simulink model "LightningModel"  (R2015a)
settings: Solver=ode23tb  StartTime=0.0  StopTime=0.04  RelTol=1e-3
libraries: powerlib x11, simulink x1
settings Model: CovSFcnEnable=off  Creator=Rodney Tan  LastModifiedBy=Rodney Tan
settings DebuggingCC: SolverPrmCheckMsg=warning

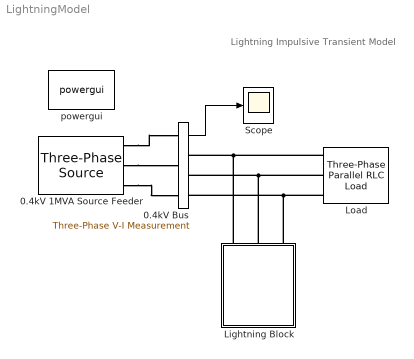
== system LightningModel ==
  note: Lightning Impulsive Transient Model
  0.4kV 1MVA Source Feeder : powerlib/Electrical Sources/Three-Phase Source  Voltage=0.4e3  PhaseAngle=0  Frequency=50  InternalConnection=Yg  SpecifyImpedance=on  Resistance=0.8929  Inductance=16.58e-3  ShortCircuitLevel=1e6  BaseVoltage=0.4e3  XRratio=7  BusType=swing  Pref=0  Qref=0  Qmin=-inf  Qmax=inf
  0.4kV Bus : powerlib/Measurements/Three-Phase V-I Measurement  VoltageMeasurement=phase-to-ground  SetLabelV=off  LabelV=Vabc  Vpu=off  VpuLL=off  CurrentMeasurement=no  SetLabelI=off  LabelI=Iabc  Ipu=off  Pbase=100e6  Vbase=500e3  OutputType=Complex  PhasorSimulation=off  PSBequivalent=0
  Lightning Block : Subsystem  mask(Lightning Model){mag=1e3, t1=0.012, R=1, L=1e-6}
      mask prompts: mag "Impulse Magnitude"; t1 "Impulse Start Time (s)"; R "Coupling Resistance (Ohms)"; L "Coupling Inductance (H)"
      mask help:
      | This lightning model simulate a 1.2/50us impulsive transient voltage defined by IEEE 1159.1 Standard. The impulsive transient is model by
      |
      | v = A*exp(-alpha*abs(t-t1))*u;
      |
      | where A is the impulse magnitude, t1 is the impulse start time, alpha is the damping factor of 14000 and u is the step function.
      mask DialogControl Container3 Prompt: Lightning Coupling
      mask Display: image('LightningBlock.jpg');
  Load : powerlib/Elements/Three-Phase Parallel RLC Load  LConnTagsString=A|B|C  Configuration=Y (grounded)  NominalVoltage=0.4e3  NominalFrequency=50  ActivePower=10e3  InductivePower=100  CapacitivePower=0  Measurements=None  LoadType=constant Z
  Scope : Scope
      settings: SampleTime=1/102400
  powergui : powerlib/powergui  Priority=1  SimulationMode=Continuous  SolverType=Tustin  SampleTime=50e-6  frequency=60  SPID=off  DisableSnubberDevices=off  DisableRonSwitches=off  DisableVfSwitches=off  SwTol=0  DisplayEquations=off  Interpol=off  methode=off  Ts=0  FunctionMessages=off  echomessages=off  HookPort=off  EnableUseOfTLC=off  x0status=blocks  frequencyindice=50  Pbase=100e6  ErrMax=1e-4  Iterations=50  UnitsV=kV  UnitsW=MW  buscounter=0  RestoreLinks=warning  ResistiveCurrentMeasurement=off  Frange=[0:2:500]  Ylog=off  Xlog=on  ShowGrid=off  save=off  variable=ZData  structure=0  ZoomFFT=off  StartTime=0.0  cycles=1  DisplayStyle=1  fundamental=60  FreqAxis=off  MaxFrequency=1000  frequencyindicesteady=1  RmsSteady=1  display=off
  wires:
  0.4kV Bus/1 -> Scope/1
  connections:
  0.4kV 1MVA Source Feeder/RConn2 -- 0.4kV Bus/LConn2
  0.4kV 1MVA Source Feeder/RConn3 -- 0.4kV Bus/LConn3
  0.4kV 1MVA Source Feeder/RConn1 -- 0.4kV Bus/LConn1
  Lightning Block/LConn2 -- Load/LConn2 -- 0.4kV Bus/RConn2
  Lightning Block/LConn1 -- Load/LConn1 -- 0.4kV Bus/RConn1
  Lightning Block/LConn3 -- Load/LConn3 -- 0.4kV Bus/RConn3

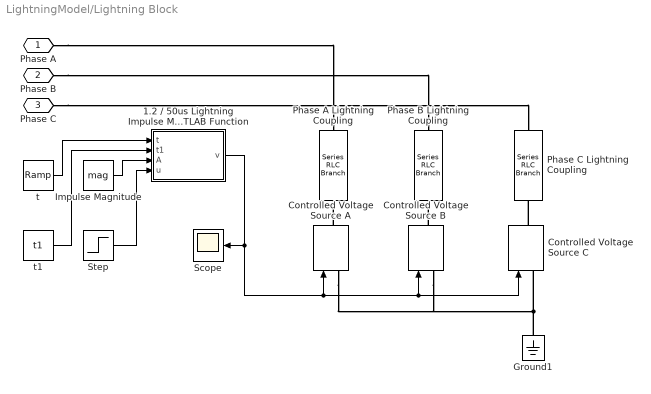
== system LightningModel/Lightning Block ==
  1.2 / 50us Lightning Impulse MATLAB Function : MATLAB Function  TreatAsAtomicUnit=on
  Controlled Voltage Source C : powerlib/Electrical Sources/Controlled Voltage Source  Initialize=on  Source_Type=DC  Amplitude=0  Phase=0  Frequency=0  Measurements=None
  Controlled Voltage Source A : powerlib/Electrical Sources/Controlled Voltage Source  Initialize=on  Source_Type=DC  Amplitude=0  Phase=0  Frequency=0  Measurements=None
  Controlled Voltage Source B : powerlib/Electrical Sources/Controlled Voltage Source  Initialize=on  Source_Type=DC  Amplitude=0  Phase=0  Frequency=0  Measurements=None
  Ground1 : powerlib/Elements/Ground  LConnTagsString=a
  Impulse Magnitude : Constant  Value=mag
  Phase A Lightning Coupling : powerlib/Elements/Series RLC Branch  LConnTagsString=__new0  RConnTagsString=__new0  BranchType=RL  Resistance=R  Inductance=L  SetiL0=off  InitialCurrent=0  Capacitance=1e-6  Setx0=off  InitialVoltage=0  Measurements=None
  Phase B Lightning Coupling : powerlib/Elements/Series RLC Branch  LConnTagsString=__new0  RConnTagsString=__new0  BranchType=RL  Resistance=R  Inductance=L  SetiL0=off  InitialCurrent=0  Capacitance=1e-6  Setx0=off  InitialVoltage=0  Measurements=None
  Phase C Lightning Coupling : powerlib/Elements/Series RLC Branch  LConnTagsString=__new0  RConnTagsString=__new0  BranchType=RL  Resistance=R  Inductance=L  SetiL0=off  InitialCurrent=0  Capacitance=1e-6  Setx0=off  InitialVoltage=0  Measurements=None
  Scope : Scope
      settings: SampleInput=on  SampleTime=1/1e6
  Step : Step  Time=t1  SampleTime=0
  t : simulink/Sources/Ramp  slope=1  start=0  X0=0
  t1 : Constant  Value=t1
  Phase A : PMIOPort  Port=1  Side=Left
  Phase B : PMIOPort  Port=2  Side=Left
  Phase C : PMIOPort  Port=3  Side=Left
  wires:
  1.2 / 50us Lightning Impulse MATLAB Function/1(v) -> Scope/1, Controlled Voltage Source A/1, Controlled Voltage Source C/1, Controlled Voltage Source B/1
  t/1 -> 1.2 / 50us Lightning Impulse MATLAB Function/1(t)
  t1/1 -> 1.2 / 50us Lightning Impulse MATLAB Function/2(t1)
  Impulse Magnitude/1 -> 1.2 / 50us Lightning Impulse MATLAB Function/3(A)
  Step/1 -> 1.2 / 50us Lightning Impulse MATLAB Function/4(u)
  connections:
  Ground1/LConn1 -- Controlled Voltage Source A/LConn1 -- Controlled Voltage Source B/LConn1 -- Controlled Voltage Source C/LConn1
  Controlled Voltage Source C/RConn1 -- Phase C Lightning Coupling/RConn1
  Controlled Voltage Source A/RConn1 -- Phase A Lightning Coupling/RConn1
  Phase A/RConn1 -- Phase A Lightning Coupling/LConn1
  Phase B/RConn1 -- Phase B Lightning Coupling/LConn1
  Controlled Voltage Source B/RConn1 -- Phase B Lightning Coupling/RConn1
  Phase C/RConn1 -- Phase C Lightning Coupling/LConn1

== matlab function LightningModel/Lightning Block/1.2 // 50us Lightning Impulse MATLAB Function ==
  data: t input; t1 input; A input; v output; u input
function v = fcn(t,t1,A,u)
alpha=14000;
v = A*exp(-alpha*abs(t-t1))*u;
